simulink model "model_test2020a"  (R2020a)
settings: Solver=FixedStepAuto  StartTime=0.0  StopTime=10.0  FixedStep=1e-3  RelTol=1e-3
InitFcn:
  | % parameters
  | M = 0.25;
  | m = .03;
  | g = 9.81;
  | R = .03;
  | l = .22;
  | 
  | k_thrust = 1.58;
  | k_momen = 0.23;
  | 
  | k_p_z = 5;
  | k_i_z = .1;
StopFcn:
  | plot3(x,y,-z);
  | xlabel('x');
  | ylabel('y');
  | zlabel('z');
  | grid on;
undefined symbols (not defined in the file or in its folder): k_i_phi, k_i_psi, k_i_tt, k_i_x, k_i_y, k_p_phi, k_p_psi, k_p_tt, k_p_x, k_p_y
libraries: simulink x4
settings Model: Creator=luand  LastModifiedBy=luand
settings DataIOCC: ReturnWorkspaceOutputs=off
settings DebuggingCC: UnconnectedInputMsg=none  UnconnectedOutputMsg=none  UnconnectedLineMsg=none
settings ModelReferenceCC: EnableRefExpFcnMdlSchedulingChecks=off
settings RTWCC: Description=Generic Real-Time Target

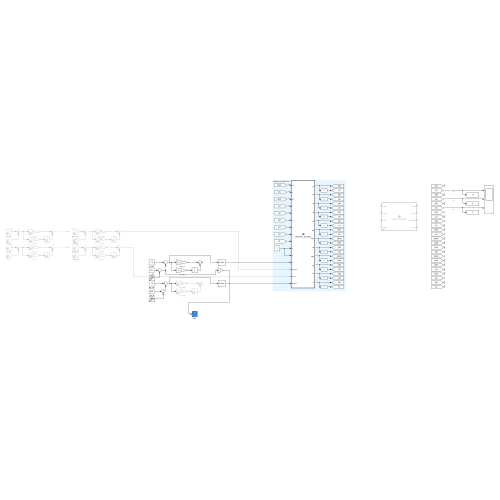
[thumbnail: Simulink's stored preview of the top-level diagram]
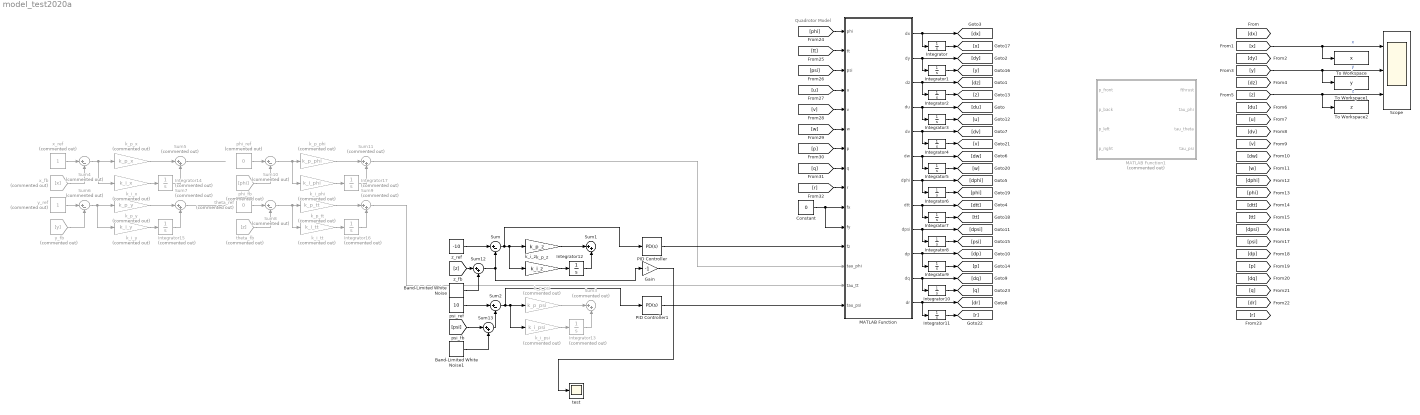
== system model_test2020a ==
  note: Quadrotor Model
  Band-Limited White Noise : simulink/Sources/Band-Limited White Noise  Cov=[0.0001]  Ts=0.1  seed=[23341]
  Band-Limited White Noise1 : simulink/Sources/Band-Limited White Noise  Cov=[0.01]  Ts=0.1  seed=[23341]
  Constant : Constant  Value=0
  Gain : Gain  Gain=-1
  Integrator{,1..12} (13 alike) : Integrator
  Integrator{13..17} (5 alike) : Integrator  Commented=on
  MATLAB Function : MATLAB Function  TreatAsAtomicUnit=on
  MATLAB Function1 : MATLAB Function  Commented=on  TreatAsAtomicUnit=on
  PID Controller : simulink/Continuous/PID Controller  Controller=PD  Form=Parallel  TimeDomain=Continuous-time  UseExternalTs=off  SampleTime=-1  IntegratorMethod=Forward Euler  ControllerParametersSource=internal  P=-0.16217268834556  I=0.00548526717818636  D=-0.299430943123664  N=1142.8279760416  UseFilter=on  TunerSelectOption=Transfer Function Based (PID Tuner App)  InitialConditionSource=internal  InitialConditionForIntegrator=0  InitialConditionForFilter=0  DifferentiatorICPrevScaledInput=0  ExternalReset=none  TrackingMode=off  Kt=1  LimitOutput=off  UpperSaturationLimit=inf  LowerSaturationLimit=-inf  LinearizeAsGain=on  AntiWindupMode=none  Kb=1  POutMin=[]  POutMax=[]  IOutMin=[]  IOutMax=[]  DOutMin=[]  DOutMax=[]  NOutMin=[]  NOutMax=[]  SumOutMin=[]  SumOutMax=[]  SaturationOutMin=[]  SaturationOutMax=[]  PParamMin=[]  PParamMax=[]  IParamMin=[]  IParamMax=[]  DParamMin=[]  DParamMax=[]  NParamMin=[]  NParamMax=[]  KbParamMin=[]  KbParamMax=[]  KtParamMin=[]  KtParamMax=[]  KbOutMin=[]  KbOutMax=[]  KtOutMin=[]  KtOutMax=[]  IntegratorOutMin=[]  IntegratorOutMax=[]  FilterOutMin=[]  FilterOutMax=[]  SumI1OutMin=[]  SumI1OutMax=[]  SumI2OutMin=[]  SumI2OutMax=[]  SumI3OutMin=[]  SumI3OutMax=[]  SumI4OutMin=[]  SumI4OutMax=[]  SumDOutMin=[]  SumDOutMax=[]  DifferentiatorOutMin=[]  DifferentiatorOutMax=[]  FilterDiffOutCoefMin=[]  FilterDiffOutCoefMax=[]  ReciprocalOutMin=[]  ReciprocalOutMax=[]  SumDenOutMin=[]  SumDenOutMax=[]  SumNumOutMin=[]  SumNumOutMax=[]  DivideOutMin=[]  DivideOutMax=[]  UdiffTsProdOutMin=[]  UdiffTsProdOutMax=[]  NTsProdOutMin=[]  NTsProdOutMax=[]  UintegralTsProdOutMin=[]  UintegralTsProdOutMax=[]  UngainTsProdOutMin=[]  UngainTsProdOutMax=[]  IntegratorContinuousStateAttributes=''  IntegratorStateMustResolveToSignalObject=off  IntegratorRTWStateStorageClass=Auto  FilterContinuousStateAttributes=''  FilterStateMustResolveToSignalObject=off  FilterRTWStateStorageClass=Auto  ParallelPVariant=InternalParameters  IdealPVariant=Disabled  IVariant=Disabled  DVariant=InternalParameters  IntegratorVariant=Disabled  SatVariant=Disabled  AWVariant=Disabled  PCopyVariant=Disabled  TRVariant=Disabled  FdbkBlocksVariant=Forward  IdealPFdbkVariant=Disabled  SatFdbkVariant=Disabled  DerivativeFilterVariant=ContFilter  NVariant=InternalParameters  NCopyVariant=Disabled  FilterICVariant=InternalICsFilter  IntegratorICVariant=Disabled  ExternalResetVariant=Disabled  TRSumVariant=Passthrough  SumFdbkVariant=Disabled  SumVariant=Sum_PD  TsampFilterVariant=InternalTs  TsampNgainVariant=Passthrough  TsampIntegralVariant=Disabled_SignalSpec
  PID Controller1 : simulink/Continuous/PID Controller  Controller=PD  Form=Parallel  TimeDomain=Continuous-time  UseExternalTs=off  SampleTime=-1  IntegratorMethod=Forward Euler  ControllerParametersSource=internal  P=0.0174840520905053  I=1  D=0.0589410393685465  N=1142.8279760416  UseFilter=on  TunerSelectOption=Transfer Function Based (PID Tuner App)  InitialConditionSource=internal  InitialConditionForIntegrator=0  InitialConditionForFilter=0  DifferentiatorICPrevScaledInput=0  ExternalReset=none  TrackingMode=off  Kt=1  LimitOutput=off  UpperSaturationLimit=inf  LowerSaturationLimit=-inf  LinearizeAsGain=on  AntiWindupMode=none  Kb=1  POutMin=[]  POutMax=[]  IOutMin=[]  IOutMax=[]  DOutMin=[]  DOutMax=[]  NOutMin=[]  NOutMax=[]  SumOutMin=[]  SumOutMax=[]  SaturationOutMin=[]  SaturationOutMax=[]  PParamMin=[]  PParamMax=[]  IParamMin=[]  IParamMax=[]  DParamMin=[]  DParamMax=[]  NParamMin=[]  NParamMax=[]  KbParamMin=[]  KbParamMax=[]  KtParamMin=[]  KtParamMax=[]  KbOutMin=[]  KbOutMax=[]  KtOutMin=[]  KtOutMax=[]  IntegratorOutMin=[]  IntegratorOutMax=[]  FilterOutMin=[]  FilterOutMax=[]  SumI1OutMin=[]  SumI1OutMax=[]  SumI2OutMin=[]  SumI2OutMax=[]  SumI3OutMin=[]  SumI3OutMax=[]  SumI4OutMin=[]  SumI4OutMax=[]  SumDOutMin=[]  SumDOutMax=[]  DifferentiatorOutMin=[]  DifferentiatorOutMax=[]  FilterDiffOutCoefMin=[]  FilterDiffOutCoefMax=[]  ReciprocalOutMin=[]  ReciprocalOutMax=[]  SumDenOutMin=[]  SumDenOutMax=[]  SumNumOutMin=[]  SumNumOutMax=[]  DivideOutMin=[]  DivideOutMax=[]  UdiffTsProdOutMin=[]  UdiffTsProdOutMax=[]  NTsProdOutMin=[]  NTsProdOutMax=[]  UintegralTsProdOutMin=[]  UintegralTsProdOutMax=[]  UngainTsProdOutMin=[]  UngainTsProdOutMax=[]  IntegratorContinuousStateAttributes=''  IntegratorStateMustResolveToSignalObject=off  IntegratorRTWStateStorageClass=Auto  FilterContinuousStateAttributes=''  FilterStateMustResolveToSignalObject=off  FilterRTWStateStorageClass=Auto  ParallelPVariant=InternalParameters  IdealPVariant=Disabled  IVariant=Disabled  DVariant=InternalParameters  IntegratorVariant=Disabled  SatVariant=Disabled  AWVariant=Disabled  PCopyVariant=Disabled  TRVariant=Disabled  FdbkBlocksVariant=Forward  IdealPFdbkVariant=Disabled  SatFdbkVariant=Disabled  DerivativeFilterVariant=ContFilter  NVariant=InternalParameters  NCopyVariant=Disabled  FilterICVariant=InternalICsFilter  IntegratorICVariant=Disabled  ExternalResetVariant=Disabled  TRSumVariant=Passthrough  SumFdbkVariant=Disabled  SumVariant=Sum_PD  TsampFilterVariant=InternalTs  TsampNgainVariant=Passthrough  TsampIntegralVariant=Disabled_SignalSpec
  Scope : Scope  NumInputPorts=3
  Sum : Sum  Inputs=|+-
  Sum1 : Sum  Inputs=|++
  Sum{4,6,8,10} (4 alike) : Sum  Commented=on  Inputs=|+-
  Sum{3,5,7,9,11} (5 alike) : Sum  Commented=on  Inputs=|++
  Sum12 : Sum  Inputs=|++
  Sum13 : Sum  Inputs=|++
  Sum2 : Sum  Inputs=|+-
  To Workspace : ToWorkspace  VariableName=x  SampleTime=-1
      settings: Save2DSignal=2-D array (concatenate along first dimension)
  To Workspace1 : ToWorkspace  VariableName=y  SampleTime=-1
      settings: Save2DSignal=2-D array (concatenate along first dimension)
  To Workspace2 : ToWorkspace  VariableName=z  SampleTime=-1
      settings: Save2DSignal=2-D array (concatenate along first dimension)
  k_i_phi : Gain  Commented=on  Gain=k_i_phi
  k_i_psi : Gain  Commented=on  Gain=k_i_psi
  k_i_tt : Gain  Commented=on  Gain=k_i_tt
  k_i_x : Gain  Commented=on  Gain=k_i_x
  k_i_y : Gain  Commented=on  Gain=k_i_y
  k_i_z : Gain  Gain=k_i_z
  k_p_phi : Gain  Commented=on  Gain=k_p_phi
  k_p_psi : Gain  Commented=on  Gain=k_p_psi
  k_p_tt : Gain  Commented=on  Gain=k_p_tt
  k_p_x : Gain  Commented=on  Gain=k_p_x
  k_p_y : Gain  Commented=on  Gain=k_p_y
  k_p_z : Gain  Gain=k_p_z
  phi_fb : From  Commented=on  GotoTag=phi
  phi_ref : Constant  Commented=on  Value=0
  psi_ref : Constant  Value=10
  test : Scope
  theta_fb : From  Commented=on  GotoTag=z
  theta_ref : Constant  Commented=on  Value=0
  x_fb : From  Commented=on  GotoTag=x
  x_ref : Constant  Commented=on
  y_fb : From  Commented=on  GotoTag=y
  y_ref : Constant  Commented=on
  z_ref : Constant  Value=-10
  wires:
  MATLAB Function/12(dr) -> Integrator11/1, [dr]
  MATLAB Function/11(dq) -> Integrator10/1, [dq]
  MATLAB Function/10(dp) -> Integrator9/1, [dp]
  MATLAB Function/9(dpsi) -> Integrator8/1, [dpsi]
  MATLAB Function/8(dtt) -> Integrator7/1, [dtt]
  MATLAB Function/7(dphi) -> Integrator6/1, [dphi]
  MATLAB Function/6(dw) -> Integrator5/1, [dw]
  MATLAB Function/5(dv) -> Integrator4/1, [dv]
  MATLAB Function/4(du) -> Integrator3/1, [du]
  MATLAB Function/3(dz) -> Integrator2/1, [dz]
  MATLAB Function/2(dy) -> Integrator1/1, [dy]
  MATLAB Function/1(dx) -> Integrator/1, [dx]
  Integrator/1 -> [x]
  Integrator1/1 -> [y]
  Integrator3/1 -> [u]
  Integrator2/1 -> [z]
  Integrator4/1 -> [v]
  Integrator5/1 -> [w]
  Integrator6/1 -> [phi]
  Integrator7/1 -> [tt]
  Integrator8/1 -> [psi]
  Integrator9/1 -> [p]
  Integrator10/1 -> [q]
  Integrator11/1 -> [r]
  [phi] -> MATLAB Function/1(phi)
  [tt] -> MATLAB Function/2(tt)
  [psi] -> MATLAB Function/3(psi)
  [u] -> MATLAB Function/4(u)
  [v] -> MATLAB Function/5(v)
  [w] -> MATLAB Function/6(w)
  [p] -> MATLAB Function/7(p)
  [x] -> Scope/1, To Workspace/1  "x"
  [y] -> Scope/2, To Workspace1/1  "y"
  [z] -> Scope/3, To Workspace2/1  "z"
  [q] -> MATLAB Function/8(q)
  [r] -> MATLAB Function/9(r)
  k_i_z/1 -> Integrator12/1
  Sum/1 -> PID Controller/1, k_p_z/1, k_i_z/1
  k_p_z/1 -> Sum1/1
  Integrator12/1 -> Sum1/2
  Integrator13/1 -> Sum3/2
  k_p_psi/1 -> Sum3/1
  psi_ref/1 -> Sum2/1
  k_i_psi/1 -> Integrator13/1
  Sum2/1 -> PID Controller1/1, k_p_psi/1, k_i_psi/1
  Integrator14/1 -> Sum5/2
  k_p_x/1 -> Sum5/1
  x_fb/1 -> Sum4/2
  x_ref/1 -> Sum4/1
  k_i_x/1 -> Integrator14/1
  Sum5/1 -> ?
  Sum4/1 -> k_p_x/1, k_i_x/1
  Integrator15/1 -> Sum7/2
  k_p_y/1 -> Sum7/1
  y_fb/1 -> Sum6/2
  y_ref/1 -> Sum6/1
  k_i_y/1 -> Integrator15/1
  Sum7/1 -> ?
  Sum6/1 -> k_p_y/1, k_i_y/1
  Sum10/1 -> k_p_phi/1, k_i_phi/1
  Sum11/1 -> MATLAB Function/13(tau_phi)
  k_i_phi/1 -> Integrator17/1
  phi_ref/1 -> Sum10/1
  phi_fb/1 -> Sum10/2
  k_p_phi/1 -> Sum11/1
  Integrator17/1 -> Sum11/2
  Sum9/1 -> MATLAB Function/14(tau_tt)
  Integrator16/1 -> Sum9/2
  k_p_tt/1 -> Sum9/1
  theta_fb/1 -> Sum8/2
  Sum8/1 -> k_p_tt/1, k_i_tt/1
  theta_ref/1 -> Sum8/1
  k_i_tt/1 -> Integrator16/1
  Constant/1 -> MATLAB Function/11(fy), MATLAB Function/10(fx)
  z_ref/1 -> Sum/1
  PID Controller/1 -> MATLAB Function/12(fz)
  PID Controller1/1 -> MATLAB Function/15(tau_psi)
  [z] -> Sum12/1
  Sum12/1 -> Sum/2, Gain/1
  Band-Limited White Noise/1 -> Sum12/2
  [psi] -> Sum13/1
  Sum13/1 -> Sum2/2
  Band-Limited White Noise1/1 -> Sum13/2
  Gain/1 -> test/1

== matlab function model_test2020a/MATLAB Function1 ==
  data: fthrust output; tau_phi output; tau_theta output; tau_psi output; p_front input; p_back input; p_left input; p_right input
function [fthrust, tau_phi, tau_theta, tau_psi] = Motor_dynamics(p_front, p_back, p_left, p_right)

fthrust = k_thrust*(p_front+p_back+p_left+p_right);
tau_phi = l*k_thrust*(-p_right+p_left);
tau_theta = l*k_thrust*(p_front+p_back);
tau_psi = k_momen*(-p_front-p_back+p_left+p_right);

== matlab function model_test2020a/MATLAB Function ==
  data: phi input; tt input; psi input; u input; dx output; v input; w input; p input; q input; r input; fx input; fy input; fz input; tau_phi input; tau_tt input; tau_psi input; dy output; dz output; du output; dv output; dw output; dphi output; dtt output; dpsi output; dp output; dq output; dr output
function [dx,dy,dz,du,dv,dw,dphi,dtt,dpsi,dp,dq,dr]=Dynamics_plustype(phi,tt,psi,u,v,w,p,q,r,fx,fy,fz,tau_phi,tau_tt,tau_psi)

M = 0.25;
m = .03;
g = 9.81;
R = .03;
l = .22;

Jx = .4*M*R*R+2*l*l*m;
Jy = .4*M*R*R+2*l*l*m;
Jz = .4*M*R*R+4*l*l*m;

dx = cos(tt)*cos(psi)*u+(sin(phi)*sin(tt)*cos(psi)-cos(phi)*sin(psi))*v+(cos(phi)*sin(tt)*cos(psi)+sin(phi)*sin(psi))*w;
dy = cos(tt)*sin(psi)*u+(sin(phi)*sin(tt)*sin(psi)+cos(phi)*cos(psi))*v+(cos(phi)*sin(tt)*sin(psi)-sin(phi)*cos(psi))*w;
dz = sin(tt)*u-sin(phi)*cos(tt)*v-cos(phi)*cos(tt)*w;

du = (r*v-q*w)+fx/m;
dv = (p*w-r*u)+fy/m;
dw = (q*u-p*v)+fz/m;

dphi = p+sin(phi)*tan(phi)*q+cos(phi)*tan(tt)*r;
dtt  = cos(phi)*q-sin(phi)*r;
dpsi = sin(phi)*q/cos(tt)+cos(phi)*r/cos(tt);

dp = ((Jy-Jz)*q*r+tau_phi)/Jx;
dq = ((Jz-Jx)*p*r+tau_tt)/Jy;
dr = ((Jx-Jy)*q*p+tau_psi)/Jz;
